simulink model "ControlYObservadorLevitador20241"  (R2023b)
settings: Solver=VariableStepAuto  StartTime=0.0  StopTime=inf  RelTol=1e-3
values from neighbouring files (symbols this model uses):
  A = [0 1; -0.2546 -0.3939]    [Control_discreto.m]    (also in datosPlanta_LABVIEW.mat = [0  1; -0.6429  -0.5935])
  B = [0 ; 1]    [Control_discreto.m]    (also in datosPlanta_LABVIEW.mat = [0 1])
  C = [0.2506 0]    [Control_discreto.m]    (also in datosPlanta_LABVIEW.mat = [0.6388 0])
  Kcont = place(A_c,B_c,polosCont)    [Control_discreto.m]
undefined symbols (not defined in the file or in its folder): daq
libraries: daqlib x2
settings Model: Creator=Soportedrai  LastModifiedBy=oscar

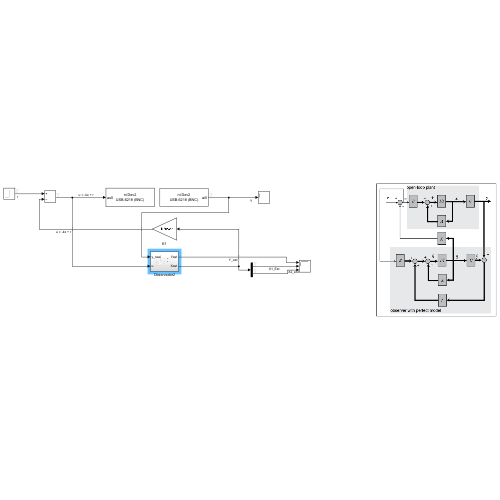
[thumbnail: Simulink's stored preview of the top-level diagram]
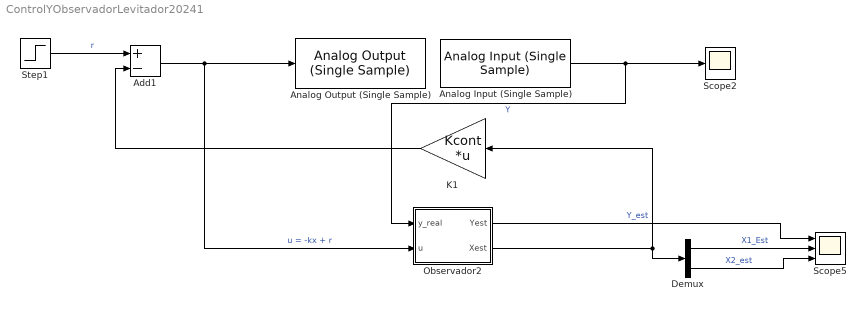
== system ControlYObservadorLevitador20241 ==
  Add1 : Sum  Inputs=+-
  Analog Input (Single Sample) : daqlib/Analog Input (Single Sample)  DeviceMenu=ni Dev2 (USB-6218 (BNC))  Device=ni Dev2 (USB-6218 (BNC))  ObjConstructor=daq.createSession('ni')  BlockSampleTime=0.1  NChannelsSelected=1  Channels=1$ai0$$Dev2$1$4$3$1$#0$ai1$$Dev2$1$4$3$1$#0$ai2$$Dev2$1$4$3$1$#0$ai3$$Dev2$1$4$3$1$#0$ai4$$Dev2$1$4$3$1$#0$ai5$$Dev2$1$4$3$1$#0$ai6$$Dev2$1$4$3$1$#0$ai7$$Dev2$1$4$3$1$#0$ai8$$Dev2$1$4$1$1$#0$ai9$$Dev2$1$4$1$1$#0$ai10$$Dev2$1$4$1$1$#0$ai11$$Dev2$1$4$1$1$#0$ai12$$Dev2$1$4$1$1$#0$ai13$$Dev2$1$4$1$1$#0$ai14$$Dev2$1$4$1$1$#0$ai15$$Dev2$1$4$1$1$#0$ai16$$Dev2$1$4$3$1$#0$ai17$$Dev2$1$4$3$1$#0$ai18$$Dev2$1$4$3$1$#0$ai19$$Dev2$1$4$3$1$#0$ai20$$Dev2$1$4$3$1$#0$ai21$$Dev2$1$4$3$1$#0$ai22$$Dev2$1$4$3$1$#0$ai23$$Dev2$1$4$3$1$#0$ai24$$Dev2$1$4$1$1$#0$ai25$$Dev2$1$4$1$1$#0$ai26$$Dev2$1$4$1$1$#0$ai27$$Dev2$1$4$1$1$#0$ai28$$Dev2$1$4$1$1$#0$ai29$$Dev2$1$4$1$1$#0$ai30$$Dev2$1$4$1$1$#0$ai31$$Dev2$1$4$1$1$#  NPorts=1 per channel  OutputTimestamp=off
  Analog Output (Single Sample) : daqlib/Analog Output (Single Sample)  DeviceMenu=ni Dev2 (USB-6218 (BNC))  Device=ni Dev2 (USB-6218 (BNC))  ObjConstructor=daq.createSession('ni')  NChannelsSelected=1  Channels=1$ao0$$Dev2$1$1$N/A$#0$ao1$$Dev2$1$1$N/A$#  NPorts=1 per channel  BlockSampleTime=0.1
  Demux : Demux  Outputs=2
  K1 : Gain  Gain=Kcont  Multiplication=Matrix(K*u) (u vector)
  Observador2 : Subsystem
  Scope2 : Scope
  Scope5 : Scope  NumInputPorts=3
  Step1 : Step  Time=0  After=0  SampleTime=0
  wires:
  Analog Input (Single Sample)/1 -> Observador2/1(y_real), Scope2/1  "Y"
  Add1/1 -> Observador2/2(u), Analog Output (Single Sample)/1  "u = -kx + r"
  Step1/1 -> Add1/1  "r"
  K1/1 -> Add1/2
  Observador2/1(Yest) -> Scope5/1  "Y_est"
  Observador2/2(Xest) -> Demux/1, K1/1
  Demux/1 -> Scope5/2  "X1_Est"
  Demux/2 -> Scope5/3  "X2_est"

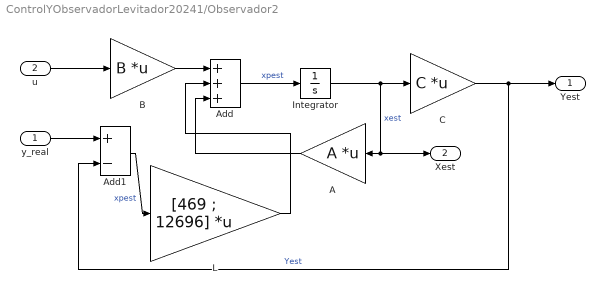
== system ControlYObservadorLevitador20241/Observador2 ==
  y_real : Inport
  u : Inport  Port=2
  A : Gain  Gain=A  Multiplication=Matrix(K*u) (u vector)
  Add : Sum  Inputs=+++
  Add1 : Sum  Inputs=+-
  B : Gain  Gain=B  Multiplication=Matrix(K*u) (u vector)
  C : Gain  Gain=C  Multiplication=Matrix(K*u) (u vector)
  Integrator : Integrator
  L : Gain  Gain=[469 ; 12696]  Multiplication=Matrix(K*u) (u vector)
  Yest : Outport
  Xest : Outport  Port=2
  wires:
  L/1 -> Add/2
  Add1/1 -> L/1  "xpest"
  y_real/1 -> Add1/1
  u/1 -> B/1
  B/1 -> Add/1
  A/1 -> Add/3
  C/1 -> Add1/2, Yest/1  "Yest"
  Integrator/1 -> Xest/1, A/1, C/1  "xest"
  Add/1 -> Integrator/1  "xpest"
